simulink model "PLL"  (R2024a)
settings: Solver=VariableStepAuto  StartTime=0.0  StopTime=10.0  RelTol=1e-3
undefined symbols (not defined in the file or in its folder): DiscIntNeverNeededParam
settings Model: Creator=Lenovo  LastModifiedBy=Lenovo

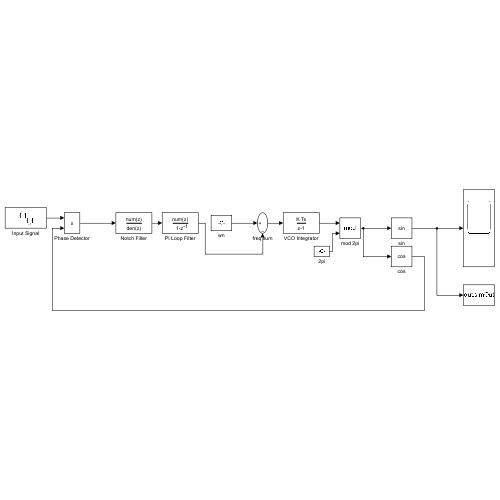
[thumbnail: Simulink's stored preview of the top-level diagram]
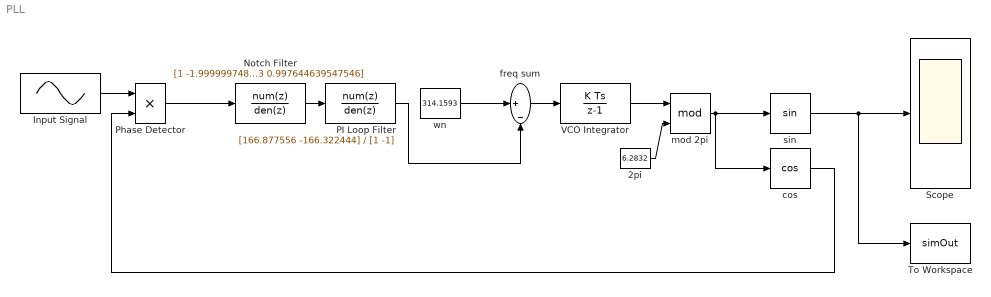
== system PLL ==
  2pi : Constant  Value=6.2832
  Input Signal : Sin  Frequency=314.1593  SampleTime=2e-05
  Notch Filter : DiscreteFilter  Numerator=[1 -1.99999974867259 1.00015766234301]  Denominator=[1 -1.99748672587713 0.997644639547546]  SampleTime=2e-05
  PI Loop Filter : DiscreteFilter  Numerator=[166.877556 -166.322444]  Denominator=[1 -1]  SampleTime=2e-05
  Phase Detector : Product
  Scope : Scope
  To Workspace : ToWorkspace  VariableName=simOut  SaveFormat=Structure With Time  SampleTime=-1
  VCO Integrator : DiscreteIntegrator  SampleTime=2e-05  ICPrevOutput=DiscIntNeverNeededParam  ICPrevScaledInput=DiscIntNeverNeededParam
  cos : Trigonometry  Operator=cos
  freq sum : Sum  Inputs=|+-
  mod 2pi : Math  Operator=mod
  sin : Trigonometry
  wn : Constant  Value=314.1593
  wires:
  Input Signal/1 -> Phase Detector/1
  cos/1 -> Phase Detector/2
  Phase Detector/1 -> Notch Filter/1
  Notch Filter/1 -> PI Loop Filter/1
  wn/1 -> freq sum/1
  PI Loop Filter/1 -> freq sum/2
  freq sum/1 -> VCO Integrator/1
  VCO Integrator/1 -> mod 2pi/1
  2pi/1 -> mod 2pi/2
  mod 2pi/1 -> sin/1, cos/1
  sin/1 -> Scope/1, To Workspace/1
